simulink model "pHCont"  (R2021b)
settings: Solver=ode3  StartTime=0.0  StopTime=2500  FixedStep=0.5  RelTol=1e-3  EnableMultiTasking=on
settings Model: SimulationMode=accelerator  Creator=ismt  LastModifiedBy=ismt
settings SolverCC: AlgebraicLoopSolver=TrustRegion
settings DataIOCC: SaveFormat=Array  SignalLoggingSaveFormat=ModelDataLogs  ReturnWorkspaceOutputs=off
settings OptimizationCC: ExpressionDepthLimit=2147483647  InitFltsAndDblsToZero=on  LifeSpan=inf
settings DebuggingCC: UnderspecifiedInitializationDetection=Classic  MergeDetectMultiDrivingBlocksExec=none  SolverPrmCheckMsg=warning  FcnCallInpInsideContextMsg=warning  StateNameClashWarn=warning  SFUnexpectedBacktrackingDiag=warning  SFNoUnconditionalDefaultTransitionDiag=warning  SFExecutionAtInitializationDiag=none  SFMachineParentedDataDiag=warning  ArithmeticOperatorsInVariantConditions=warning
settings HardwareCC: ProdBitPerPointer=32  ProdBitPerSizeT=32  ProdBitPerPtrDiffT=32  ProdLargestAtomicFloat=None  ProdIntDivRoundTo=Undefined  ProdEndianess=Unspecified  ProdWordSize=32  ProdHWDeviceType=32-bit Generic
settings ModelReferenceCC: PropagateSignalLabelsOutOfModel=off
settings CodeAppCC: StateflowObjectComments=on
settings GRTTargetCC: TargetLangStandard=C89/C90 (ANSI)  CombineOutputUpdateFcns=off  GRTInterface=on
settings ConfigComp: CovMetricSettings=dw  CovSaveCumulativeToWorkspaceVar=on  CovSaveSingleToWorkspaceVar=on

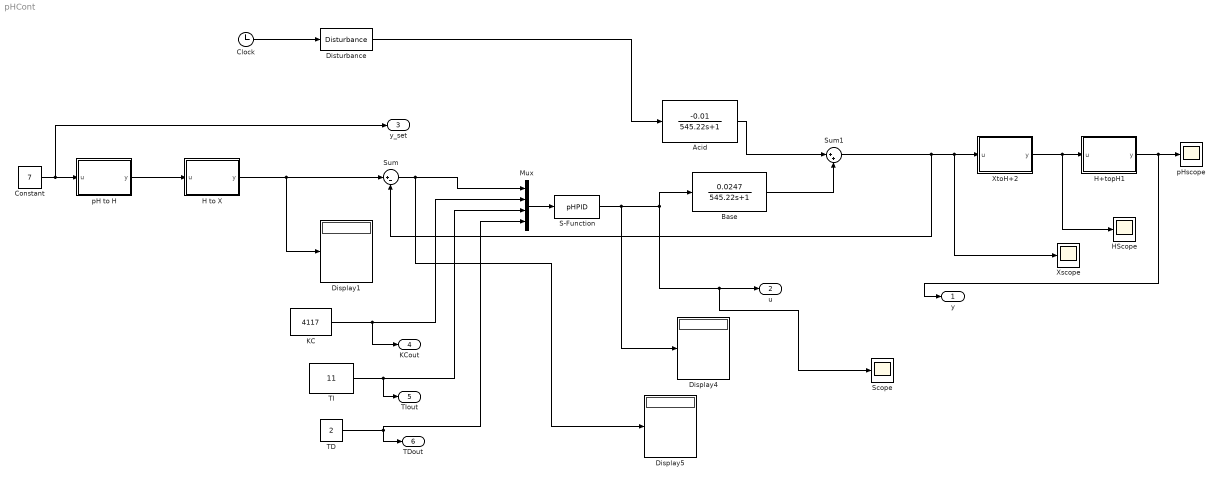
== system pHCont ==
  Acid : TransferFcn  Numerator=[-0.01]  Denominator=[545.22 1]
  Base : TransferFcn  Numerator=[0.0247]  Denominator=[545.22 1]
  Clock : Clock
  Constant : Constant  Value=7  SampleTime=-1
  Display1 : Display
  Display4 : Display
  Display5 : Display
  Disturbance : MATLABFcn  MATLABFcn=Disturbance
  H to X : MATLAB Function  TreatAsAtomicUnit=on
  H+topH1 : MATLAB Function  TreatAsAtomicUnit=on
  HScope : Scope
  KC : Constant  Value=4117  SampleTime=-1
  Mux : Mux
  S-Function : S-Function  FunctionName=pHPID  SFunctionDeploymentMode=off  EnableBusSupport=off
  Scope : Scope
  Sum : Sum  Inputs=|+-
  Sum1 : Sum  Inputs=|++
  TD : Constant  Value=2  SampleTime=-1
  TI : Constant  Value=11  SampleTime=-1
  Xscope : Scope
  XtoH+2 : MATLAB Function  TreatAsAtomicUnit=on
  pH to H : MATLAB Function  TreatAsAtomicUnit=on
  pHscope : Scope
  y : Outport
  u : Outport  Port=2
  y_set : Outport  Port=3
  KCout : Outport  Port=4
  TIout : Outport  Port=5
  TDout : Outport  Port=6
  wires:
  Sum/1 -> Display5/1, Mux/1
  KC/1 -> Mux/2, KCout/1
  TI/1 -> Mux/3, TIout/1
  TD/1 -> Mux/4, TDout/1
  Mux/1 -> S-Function/1
  S-Function/1 -> Display4/1, Base/1, Scope/1, u/1
  Disturbance/1 -> Acid/1
  Constant/1 -> y_set/1, pH to H/1(u)
  Acid/1 -> Sum1/1
  Base/1 -> Sum1/2
  H+topH1/1(y) -> y/1, pHscope/1
  pH to H/1(y) -> H to X/1(u)
  H to X/1(y) -> Display1/1, Sum/1
  XtoH+2/1(y) -> HScope/1, H+topH1/1(u)
  Sum1/1 -> Sum/2, Xscope/1, XtoH+2/1(u)
  Clock/1 -> Disturbance/1

== matlab function pHCont/pH to H ==
  data: u input; y output
function y = fcn(u)

y = 10^(-u);
end

== matlab function pHCont/H+topH1 ==
  data: u input; y output
function y = fcn(u)

y = -log10(u);
end

== matlab function pHCont/H to X ==
  data: u input; y output
function y = fcn(u)

y = ((10^(-14))-(u^2))/u;
end

== matlab function pHCont/XtoH+2 ==
  data: u input; y output
function y = fcn(u)

y = sqrt(((u^2)/4) + 10^(-14))-(u/2);
end
